simulink model "CoME_DemCoord"  (R2016b)
settings: configuration reference "CodeGenConfigSet" (kept outside this file)
values from neighbouring files (symbols this model uses):
  CoME_stNReqESS_C = Calibration.Parameter    [init_CoME_DemCoord.m]    (also in init_CoME_DemCoord_SIL.m = Simulink.Parameter)
  CoME_stNReqTS_C = Calibration.Parameter    [init_CoME_DemCoord.m]    (also in init_CoME_DemCoord_SIL.m = Simulink.Parameter)
  CoME_stNReqTSAC_C = Calibration.Parameter    [init_CoME_DemCoord.m]    (also in init_CoME_DemCoord_SIL.m = Simulink.Parameter)
  CoME_stNReqVehMot_C = Calibration.Parameter    [init_CoME_DemCoord.m]    (also in init_CoME_DemCoord_SIL.m = Simulink.Parameter)
  COME_STNSETP_UNFLT = fi(1,State_uint8)    [init_CoME_DemCoord.m]    (also in init_CoME_DemCoord_SIL.m)
  ENG_N_ZERO = fi(0,EngSpeed_rpm)    [init_CoME_DemCoord.m]    (also in init_CoME_DemCoord_SIL.m)
libraries: CXLib x4
settings Model: Creator=Colin  LastModifiedBy=Administrator
settings ConfigSetRef: SourceLocation=Base Workspace

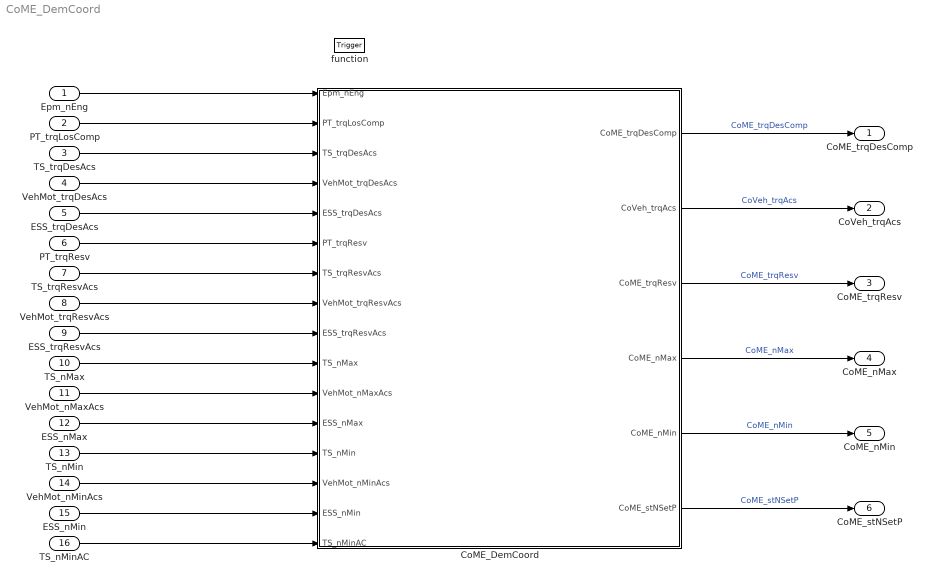
== system CoME_DemCoord ==
  Epm_nEng : Inport  Tag=rpm  Description=Engine speed  OutMin=0  OutMax=6000  OutDataTypeStr=EngSpeed_rpm
  PT_trqLosComp : Inport  Tag=Nm  Description=Torque loss of the power train  Port=2  OutMin=-3000  OutMax=3000  OutDataTypeStr=Trq_Nm
  TS_trqDesAcs : Inport  Tag=Nm  Description=Desired Torque demand of the thermal system  Port=3  OutMin=-3000  OutMax=3276.7  OutDataTypeStr=Trq_Nm
  VehMot_trqDesAcs : Inport  Tag=Nm  Description=Required engine speed of Vehicle Motion acsessories  Port=4  OutMin=-3000  OutMax=3000  OutDataTypeStr=Trq_Nm
  ESS_trqDesAcs : Inport  Tag=Nm  Description=Torque request from Electrical Supply System  Port=5  OutMin=-3000  OutMax=3276.7  OutDataTypeStr=Trq_Nm
  PT_trqResv : Inport  Tag=Nm  Description=torque reserve of the drive train  Port=6  OutMin=-3000  OutMax=3000  OutDataTypeStr=Trq_Nm
  TS_trqResvAcs : Inport  Tag=Nm  Description=Torque reserve of the thermal system  Port=7  OutMin=-3000  OutMax=3276.7  OutDataTypeStr=Trq_Nm
  VehMot_trqResvAcs : Inport  Tag=Nm  Description=Demanded engine speed reserve by acsessories of Vehicle Motion  Port=8  OutMin=-3000  OutMax=3000  OutDataTypeStr=Trq_Nm
  ESS_trqResvAcs : Inport  Tag=Nm  Description=Torque reserve due to on-board electrical system  Port=9  OutMin=-3000  OutMax=3276.7  OutDataTypeStr=Trq_Nm
  TS_nMax : Inport  Tag=rpm  Description=Highest engine speed requested by the thermal system  Port=10  OutMin=-12000  OutMax=12000  OutDataTypeStr=EngSpeed_rpm
  VehMot_nMaxAcs : Inport  Tag=rpm  Description=Maximum engine speed demand by accessories of Vehicle Motion  Port=11  OutMin=-12000  OutMax=12000  OutDataTypeStr=EngSpeed_rpm
  ESS_nMax : Inport  Tag=rpm  Description=Max. engine speed request from Electrical Supply System  Port=12  OutMin=-6000  OutMax=6000  OutDataTypeStr=EngSpeed_rpm
  TS_nMin : Inport  Tag=rpm  Description=Lowest engine speed requested by the thermal system  Port=13  OutMin=-12000  OutMax=12000  OutDataTypeStr=EngSpeed_rpm
  VehMot_nMinAcs : Inport  Tag=rpm  Description=Minimum engine speed demand by accessories of Vehicle Motion  Port=14  OutMin=-12000  OutMax=12000  OutDataTypeStr=EngSpeed_rpm
  ESS_nMin : Inport  Tag=rpm  Description=Min. engine speed request from Electrical Supply System  Port=15  OutMin=-6000  OutMax=6000  OutDataTypeStr=EngSpeed_rpm
  TS_nMinAC : Inport  Tag=rpm  Description=idle speed request  Port=16  OutMin=-12000  OutMax=12000  OutDataTypeStr=EngSpeed_rpm
  function : TriggerPort  TriggerType=function-call  VariantControl=Variant
  CoME_DemCoord : Subsystem  RTWFcnName=CoME_DemCoord_Co  RTWFileName=CoME_DemCoord
      settings: RTWSystemCode=Nonreusable function  RTWFcnNameOpts=User specified  RTWFileNameOpts=User specified
  CoME_trqDesComp : Outport  Tag=Nm  Description=Application parameter for torque demand of mechanical co-ordinator  OutMin=-3000  OutMax=3000  OutDataTypeStr=Trq_Nm
  CoVeh_trqAcs : Outport  Tag=Nm  Description=message for demand of accessories  Port=2  OutMin=-3276.8  OutMax=3276.7  OutDataTypeStr=Trq_Nm
  CoME_trqResv : Outport  Tag=Nm  Description=Reserve torque demand of mechanical co-ordinator  Port=3  OutMin=-3000  OutMax=3276.7  OutDataTypeStr=Trq_Nm
  CoME_nMax : Outport  Tag=rpm  Description=Maximum engine speed limit of accessories  Port=4  OutMin=-12000  OutMax=12000  OutDataTypeStr=EngSpeed_rpm
  CoME_nMin : Outport  Tag=rpm  Description=Minimum low-idle speed requirement of accessories  Port=5  OutMin=-12000  OutMax=12000  OutDataTypeStr=EngSpeed_rpm
  CoME_stNSetP : Outport  Description=Status: Nature of low-idle speed increase  Port=6  OutMin=0  OutMax=255  OutDataTypeStr=State_uint8
  wires:
  CoME_DemCoord/1(CoME_trqDesComp) -> CoME_trqDesComp/1  "CoME_trqDesComp"
  CoME_DemCoord/2(CoVeh_trqAcs) -> CoVeh_trqAcs/1  "CoVeh_trqAcs"
  CoME_DemCoord/3(CoME_trqResv) -> CoME_trqResv/1  "CoME_trqResv"
  CoME_DemCoord/4(CoME_nMax) -> CoME_nMax/1  "CoME_nMax"
  CoME_DemCoord/5(CoME_nMin) -> CoME_nMin/1  "CoME_nMin"
  CoME_DemCoord/6(CoME_stNSetP) -> CoME_stNSetP/1  "CoME_stNSetP"
  Epm_nEng/1 -> CoME_DemCoord/1(Epm_nEng)
  TS_nMinAC/1 -> CoME_DemCoord/16(TS_nMinAC)
  ESS_nMin/1 -> CoME_DemCoord/15(ESS_nMin)
  VehMot_nMinAcs/1 -> CoME_DemCoord/14(VehMot_nMinAcs)
  TS_nMin/1 -> CoME_DemCoord/13(TS_nMin)
  PT_trqLosComp/1 -> CoME_DemCoord/2(PT_trqLosComp)
  TS_trqDesAcs/1 -> CoME_DemCoord/3(TS_trqDesAcs)
  VehMot_trqDesAcs/1 -> CoME_DemCoord/4(VehMot_trqDesAcs)
  ESS_trqDesAcs/1 -> CoME_DemCoord/5(ESS_trqDesAcs)
  PT_trqResv/1 -> CoME_DemCoord/6(PT_trqResv)
  TS_trqResvAcs/1 -> CoME_DemCoord/7(TS_trqResvAcs)
  VehMot_trqResvAcs/1 -> CoME_DemCoord/8(VehMot_trqResvAcs)
  ESS_trqResvAcs/1 -> CoME_DemCoord/9(ESS_trqResvAcs)
  TS_nMax/1 -> CoME_DemCoord/10(TS_nMax)
  VehMot_nMaxAcs/1 -> CoME_DemCoord/11(VehMot_nMaxAcs)
  ESS_nMax/1 -> CoME_DemCoord/12(ESS_nMax)

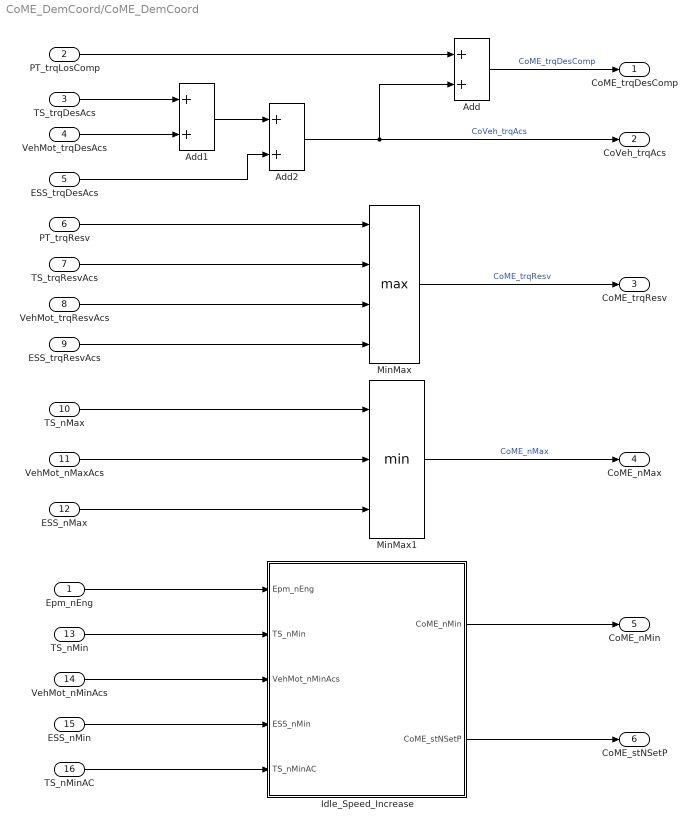
== system CoME_DemCoord/CoME_DemCoord ==
  Epm_nEng : Inport
  PT_trqLosComp : Inport  Port=2
  TS_trqDesAcs : Inport  Port=3
  VehMot_trqDesAcs : Inport  Port=4
  ESS_trqDesAcs : Inport  Port=5
  PT_trqResv : Inport  Port=6
  TS_trqResvAcs : Inport  Port=7
  VehMot_trqResvAcs : Inport  Port=8
  ESS_trqResvAcs : Inport  Port=9
  TS_nMax : Inport  Port=10
  VehMot_nMaxAcs : Inport  Port=11
  ESS_nMax : Inport  Port=12
  TS_nMin : Inport  Port=13
  VehMot_nMinAcs : Inport  Port=14
  ESS_nMin : Inport  Port=15
  TS_nMinAC : Inport  Port=16
  Add : Sum  InputSameDT=on
  Add1 : Sum  InputSameDT=on
  Add2 : Sum  InputSameDT=on
  "Idle_Speed_Increase " : Subsystem
  MinMax : MinMax  Function=max  Inputs=4  InputSameDT=on
  MinMax1 : MinMax  Inputs=3  InputSameDT=on
  CoME_trqDesComp : Outport
  CoVeh_trqAcs : Outport  Port=2
  CoME_trqResv : Outport  Port=3
  CoME_nMax : Outport  Port=4
  CoME_nMin : Outport  Port=5
  CoME_stNSetP : Outport  Port=6
  wires:
  TS_nMax/1 -> MinMax1/1
  MinMax1/1 -> CoME_nMax/1  "CoME_nMax"
  "Idle_Speed_Increase "/1(CoME_nMin) -> CoME_nMin/1
  TS_trqDesAcs/1 -> Add1/1
  TS_trqResvAcs/1 -> MinMax/2
  VehMot_nMaxAcs/1 -> MinMax1/2
  Add/1 -> CoME_trqDesComp/1  "CoME_trqDesComp"
  PT_trqResv/1 -> MinMax/1
  ESS_trqResvAcs/1 -> MinMax/4
  VehMot_trqResvAcs/1 -> MinMax/3
  ESS_trqDesAcs/1 -> Add2/2
  Add2/1 -> CoVeh_trqAcs/1, Add/2  "CoVeh_trqAcs"
  MinMax/1 -> CoME_trqResv/1  "CoME_trqResv"
  ESS_nMax/1 -> MinMax1/3
  "Idle_Speed_Increase "/2(CoME_stNSetP) -> CoME_stNSetP/1
  Add1/1 -> Add2/1
  PT_trqLosComp/1 -> Add/1
  VehMot_trqDesAcs/1 -> Add1/2
  ESS_nMin/1 -> "Idle_Speed_Increase "/4(ESS_nMin)
  TS_nMinAC/1 -> "Idle_Speed_Increase "/5(TS_nMinAC)
  TS_nMin/1 -> "Idle_Speed_Increase "/2(TS_nMin)
  Epm_nEng/1 -> "Idle_Speed_Increase "/1(Epm_nEng)
  VehMot_nMinAcs/1 -> "Idle_Speed_Increase "/3(VehMot_nMinAcs)

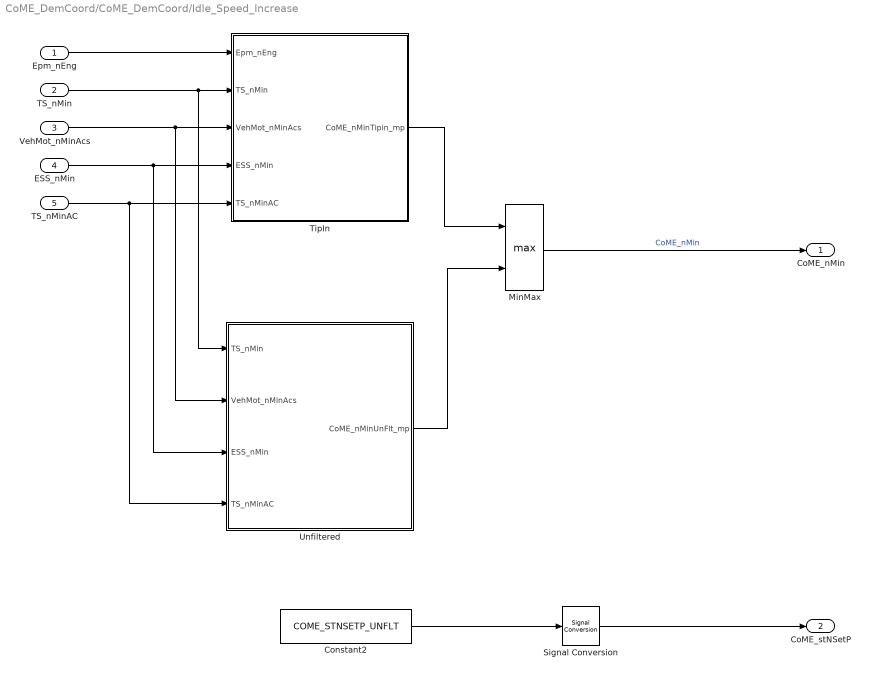
== system CoME_DemCoord/CoME_DemCoord/Idle_Speed_Increase  ==
  Epm_nEng : Inport
  TS_nMin : Inport  Port=2
  VehMot_nMinAcs : Inport  Port=3
  ESS_nMin : Inport  Port=4
  TS_nMinAC : Inport  Port=5
  Constant2 : Constant  Value=COME_STNSETP_UNFLT  OutDataTypeStr=State_uint8
  MinMax : MinMax  Function=max  Inputs=2  InputSameDT=on
  Signal Conversion : SignalConversion  OverrideOpt=off
  TipIn : Subsystem
  Unfiltered : Subsystem
  CoME_nMin : Outport
  CoME_stNSetP : Outport  Port=2
  wires:
  TS_nMinAC/1 -> Unfiltered/4(TS_nMinAC), TipIn/5(TS_nMinAC)
  Unfiltered/1(CoME_nMinUnFlt_mp) -> MinMax/2
  TipIn/1(CoME_nMinTipin_mp) -> MinMax/1
  VehMot_nMinAcs/1 -> Unfiltered/2(VehMot_nMinAcs), TipIn/3(VehMot_nMinAcs)
  ESS_nMin/1 -> Unfiltered/3(ESS_nMin), TipIn/4(ESS_nMin)
  TS_nMin/1 -> Unfiltered/1(TS_nMin), TipIn/2(TS_nMin)
  MinMax/1 -> CoME_nMin/1  "CoME_nMin"
  Constant2/1 -> Signal Conversion/1
  Epm_nEng/1 -> TipIn/1(Epm_nEng)
  Signal Conversion/1 -> CoME_stNSetP/1

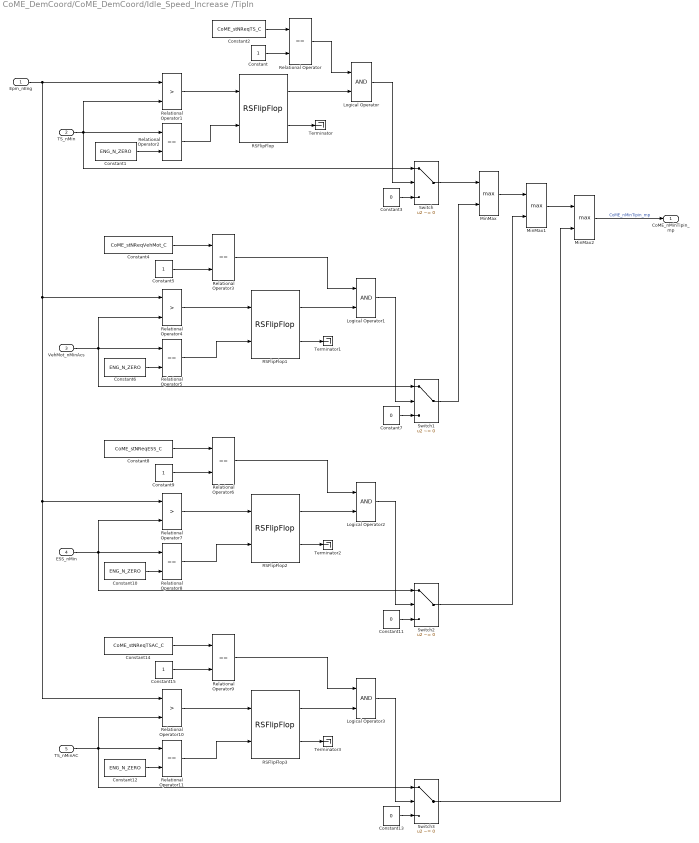
== system CoME_DemCoord/CoME_DemCoord/Idle_Speed_Increase /TipIn ==
  Epm_nEng : Inport
  TS_nMin : Inport  Port=2
  VehMot_nMinAcs : Inport  Port=3
  ESS_nMin : Inport  Port=4
  TS_nMinAC : Inport  Port=5
  Constant{,5,9,15} (4 alike) : Constant  OutDataTypeStr=Inherit: Inherit via back propagation
  Constant{1,6,10,12} (4 alike) : Constant  Value=ENG_N_ZERO  OutDataTypeStr=EngSpeed_rpm
  Constant{3,7,11,13} (4 alike) : Constant  Value=0  OutDataTypeStr=Inherit: Inherit via back propagation
  Constant14 : Constant  Value=CoME_stNReqTSAC_C
  Constant2 : Constant  Value=CoME_stNReqTS_C
  Constant4 : Constant  Value=CoME_stNReqVehMot_C
  Constant8 : Constant  Value=CoME_stNReqESS_C
  Logical Operator{,1..3} (4 alike) : Logic  OutDataTypeStr=boolean
  MinMax : MinMax  Function=max  Inputs=2  InputSameDT=on
  MinMax1 : MinMax  Function=max  Inputs=2  InputSameDT=on
  MinMax2 : MinMax  Function=max  Inputs=2  InputSameDT=on
  RSFlipFlop{,1..3} (4 alike) : CXLib/RSFlipFlop
  Relational Operator{,2..3,5..6,8..9,11} (8 alike) : RelationalOperator  Operator===  OutDataTypeStr=boolean  RndMeth=Simplest  InputSameDT=on
  Relational Operator{1,4,7,10} (4 alike) : RelationalOperator  Operator=>  OutDataTypeStr=boolean  RndMeth=Simplest  InputSameDT=on
  Switch{,1..3} (4 alike) : Switch  Criteria=u2 ~= 0  InputSameDT=on
  Terminator{,1..3} (4 alike) : Terminator
  CoME_nMinTipin_mp : Outport
  wires:
  Constant2/1 -> Relational Operator/1
  Constant/1 -> Relational Operator/2
  RSFlipFlop/2 -> Terminator/1
  RSFlipFlop/1 -> Logical Operator/2
  Relational Operator/1 -> Logical Operator/1
  Relational Operator1/1 -> RSFlipFlop/1
  Relational Operator2/1 -> RSFlipFlop/2
  Constant1/1 -> Relational Operator2/2
  TS_nMin/1 -> Switch/1, Relational Operator2/1, Relational Operator1/2
  Logical Operator/1 -> Switch/2
  Constant3/1 -> Switch/3
  Constant4/1 -> Relational Operator3/1
  Constant5/1 -> Relational Operator3/2
  RSFlipFlop1/1 -> Logical Operator1/2
  Relational Operator3/1 -> Logical Operator1/1
  Relational Operator4/1 -> RSFlipFlop1/1
  Relational Operator5/1 -> RSFlipFlop1/2
  Constant6/1 -> Relational Operator5/2
  VehMot_nMinAcs/1 -> Switch1/1, Relational Operator4/2, Relational Operator5/1
  Constant7/1 -> Switch1/3
  Logical Operator1/1 -> Switch1/2
  RSFlipFlop1/2 -> Terminator1/1
  Switch/1 -> MinMax/1
  Switch1/1 -> MinMax/2
  Constant8/1 -> Relational Operator6/1
  Constant9/1 -> Relational Operator6/2
  RSFlipFlop2/1 -> Logical Operator2/2
  Relational Operator6/1 -> Logical Operator2/1
  Relational Operator7/1 -> RSFlipFlop2/1
  Relational Operator8/1 -> RSFlipFlop2/2
  Constant10/1 -> Relational Operator8/2
  ESS_nMin/1 -> Switch2/1, Relational Operator7/2, Relational Operator8/1
  Constant11/1 -> Switch2/3
  Logical Operator2/1 -> Switch2/2
  RSFlipFlop2/2 -> Terminator2/1
  Epm_nEng/1 -> Relational Operator1/1, Relational Operator4/1, Relational Operator7/1, Relational Operator10/1
  Constant14/1 -> Relational Operator9/1
  Constant15/1 -> Relational Operator9/2
  RSFlipFlop3/1 -> Logical Operator3/2
  Relational Operator9/1 -> Logical Operator3/1
  Relational Operator10/1 -> RSFlipFlop3/1
  Relational Operator11/1 -> RSFlipFlop3/2
  Constant12/1 -> Relational Operator11/2
  TS_nMinAC/1 -> Relational Operator11/1, Relational Operator10/2, Switch3/1
  Constant13/1 -> Switch3/3
  Logical Operator3/1 -> Switch3/2
  RSFlipFlop3/2 -> Terminator3/1
  MinMax/1 -> MinMax1/1
  MinMax1/1 -> MinMax2/1
  Switch2/1 -> MinMax1/2
  Switch3/1 -> MinMax2/2
  MinMax2/1 -> CoME_nMinTipin_mp/1  "CoME_nMinTipin_mp"

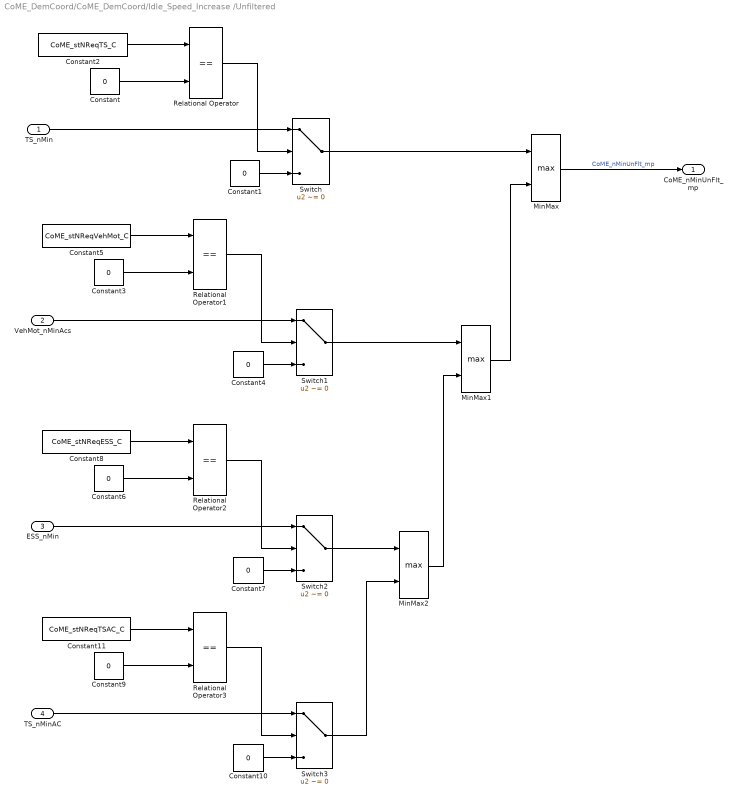
== system CoME_DemCoord/CoME_DemCoord/Idle_Speed_Increase /Unfiltered ==
  TS_nMin : Inport
  VehMot_nMinAcs : Inport  Port=2
  ESS_nMin : Inport  Port=3
  TS_nMinAC : Inport  Port=4
  Constant{,1,3..4,6..7,9..10} (8 alike) : Constant  Value=0  OutDataTypeStr=Inherit: Inherit via back propagation
  Constant11 : Constant  Value=CoME_stNReqTSAC_C
  Constant2 : Constant  Value=CoME_stNReqTS_C
  Constant5 : Constant  Value=CoME_stNReqVehMot_C
  Constant8 : Constant  Value=CoME_stNReqESS_C
  MinMax : MinMax  Function=max  Inputs=2  InputSameDT=on
  MinMax1 : MinMax  Function=max  Inputs=2  InputSameDT=on
  MinMax2 : MinMax  Function=max  Inputs=2  InputSameDT=on
  Relational Operator{,1..3} (4 alike) : RelationalOperator  Operator===  OutDataTypeStr=boolean  RndMeth=Simplest  InputSameDT=on
  Switch{,1..3} (4 alike) : Switch  Criteria=u2 ~= 0  InputSameDT=on
  CoME_nMinUnFlt_mp : Outport
  wires:
  Constant/1 -> Relational Operator/2
  Constant2/1 -> Relational Operator/1
  Relational Operator/1 -> Switch/2
  TS_nMin/1 -> Switch/1
  Constant1/1 -> Switch/3
  Switch/1 -> MinMax/1
  MinMax/1 -> CoME_nMinUnFlt_mp/1  "CoME_nMinUnFlt_mp"
  Constant3/1 -> Relational Operator1/2
  Constant5/1 -> Relational Operator1/1
  Relational Operator1/1 -> Switch1/2
  VehMot_nMinAcs/1 -> Switch1/1
  Constant4/1 -> Switch1/3
  Switch1/1 -> MinMax1/1
  MinMax1/1 -> MinMax/2
  Constant6/1 -> Relational Operator2/2
  Constant8/1 -> Relational Operator2/1
  Relational Operator2/1 -> Switch2/2
  ESS_nMin/1 -> Switch2/1
  Constant7/1 -> Switch2/3
  Switch2/1 -> MinMax2/1
  MinMax2/1 -> MinMax1/2
  Constant9/1 -> Relational Operator3/2
  Constant11/1 -> Relational Operator3/1
  Relational Operator3/1 -> Switch3/2
  TS_nMinAC/1 -> Switch3/1
  Constant10/1 -> Switch3/3
  Switch3/1 -> MinMax2/2
